simulink model "CC"  (R2015b)
settings: Solver=FixedStepDiscrete  StartTime=0.0  StopTime=inf  FixedStep=CCOk_stepSize  RelTol=1e-3
undefined symbols (not defined in the file or in its folder): CCOk_stepSize
settings Model: Creator=favv5g  LastModifiedBy=nctzv8
settings ConfigSet: Description=OpenECU configuration set for code generation under RTW-EC.
settings SolverCC: PositivePriorityOrder=on
settings DataIOCC: SaveFormat=Array  SignalLoggingSaveFormat=ModelDataLogs
settings OptimizationCC: DefaultParameterBehavior=Inlined  InlineInvariantSignals=on  ExpressionDepthLimit=2147483647  StateBitsets=on  DataBitsets=on  ZeroExternalMemoryAtStartup=off  ZeroInternalMemoryAtStartup=off  NoFixptDivByZeroProtection=on  EfficientFloat2IntCast=on  OptimizeModelRefInitCode=on  LifeSpan=1
settings DebuggingCC: SaveWithParameterizedLinksMsg=none  UnderspecifiedInitializationDetection=Classic  MergeDetectMultiDrivingBlocksExec=none  SignalResolutionControl=TryResolveAllWithWarning  MultiTaskDSMMsg=warning  MultiTaskCondExecSysMsg=none  SingleTaskRateTransMsg=error  CheckMatrixSingularityMsg=warning  VectorMatrixConversionMsg=warning  FcnCallInpInsideContextMsg=UseLocalSettings  SignalLabelMismatchMsg=warning  StateNameClashWarn=warning
settings HardwareCC: ProdBitPerPointer=32  ProdLargestAtomicInteger=Long  ProdLargestAtomicFloat=Double  ProdEndianess=BigEndian  ProdWordSize=32  ProdHWDeviceType=Freescale->32-bit PowerPC  TargetIntDivRoundTo=Zero  TargetEndianess=BigEndian  TargetHWDeviceType=Freescale->32-bit PowerPC  ProdEqTarget=off
settings RTWCC: SystemTargetFile=openecu_ert.tlc  MakeCommand=make_rtw optimized_floating_point=1  TemplateMakefile=openecu_ert_r2015b_64.tmf  Description=OpenECU Platform Target (ERT, optimised floating-point code)  RetainRTWFile=on  IncludeHyperlinkInReport=on
settings CodeAppCC: ForceParamTrailComments=on  IgnoreCustomStorageClasses=off  SimulinkDataObjDesc=on  CustomSymbolStrType=$N$R$M  InsertBlockDesc=on  InternalIdentifier=Classic
settings STFCustomTargetCC: TargetLibSuffix=.a  GenerateSampleERTMain=on  ConcurrentExecutionCompliant=off  IncludeMdlTerminateFcn=off  GeneratePreprocessorConditionals=Use local settings  CombineOutputUpdateFcns=on  IncludeFileDelimiter=UseQuote  ERTCustomFileBanners=on  SupportContinuousTime=off  MATLABClassNameForMDSCustomization=Simulink.SoftwareTarget.ERTCustomization  CPPClassGenCompliant=off  GRTInterface=off  SystemTargetFile=openecu_ert.tlc
settings ERTTargetCC: GenerateSampleERTMain=on  ParMdlRefBuildCompliant=off  CompOptLevelCompliant=off  ConcurrentExecutionCompliant=off  IncludeMdlTerminateFcn=off  ERTFirstTimeCompliant=off  IncludeFileDelimiter=UseQuote  SupportNonInlinedSFcns=on  ModelStepFunctionPrototypeControlCompliant=off  CPPClassGenCompliant=off  UseToolchainInfoCompliant=off  ExtModeMexFile=noextcomm  InlinedParameterPlacement=NonHierarchical  ERTSrcFileBannerTemplate=oe_code_c_template.cgt  ERTHdrFileBannerTemplate=oe_code_h_template.cgt  ERTDataSrcFileTemplate=oe_data_c_template.cgt  ERTDataHdrFileTemplate=oe_data_h_template.cgt  ERTCustomFileTemplate=example_file_process.tlc  GlobalDataDefinition=InSeparateSourceFile  GlobalDataReference=InSeparateHeaderFile  EnableUserReplacementTypes=on

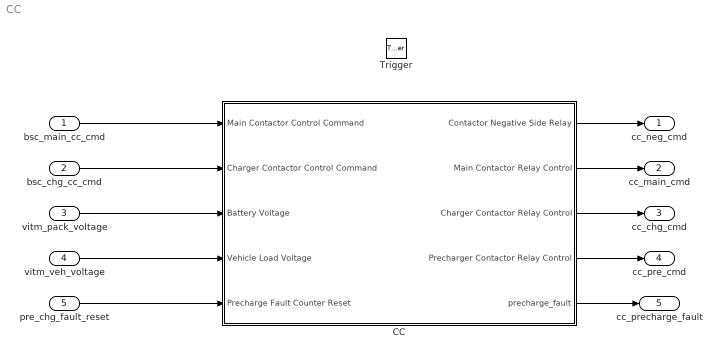
== system CC ==
  bsc_main_cc_cmd : Inport  OutDataTypeStr=boolean
  bsc_chg_cc_cmd : Inport  Port=2  OutDataTypeStr=boolean
  vitm_pack_voltage : Inport  Port=3
  vitm_veh_voltage : Inport  Port=4
  pre_chg_fault_reset : Inport  Port=5
  Trigger : TriggerPort  TriggerType=function-call  PortDimensions=1
  CC : Subsystem  TreatAsAtomicUnit=on
  cc_neg_cmd : Outport
  cc_main_cmd : Outport  Port=2
  cc_chg_cmd : Outport  Port=3
  cc_pre_cmd : Outport  Port=4
  cc_precharge_fault : Outport  Port=5
  wires:
  bsc_main_cc_cmd/1 -> CC/1(Main Contactor Control Command)
  bsc_chg_cc_cmd/1 -> CC/2(Charger Contactor Control Command)
  vitm_pack_voltage/1 -> CC/3(Battery Voltage)
  vitm_veh_voltage/1 -> CC/4(Vehicle Load Voltage)
  pre_chg_fault_reset/1 -> CC/5(Precharge Fault Counter Reset)
  CC/1("Contactor Negative Side Relay ") -> cc_neg_cmd/1
  CC/2("Main Contactor Relay Control ") -> cc_main_cmd/1
  CC/3(Charger Contactor Relay Control) -> cc_chg_cmd/1
  CC/4("Precharger Contactor Relay Control ") -> cc_pre_cmd/1
  CC/5(precharge_fault) -> cc_precharge_fault/1

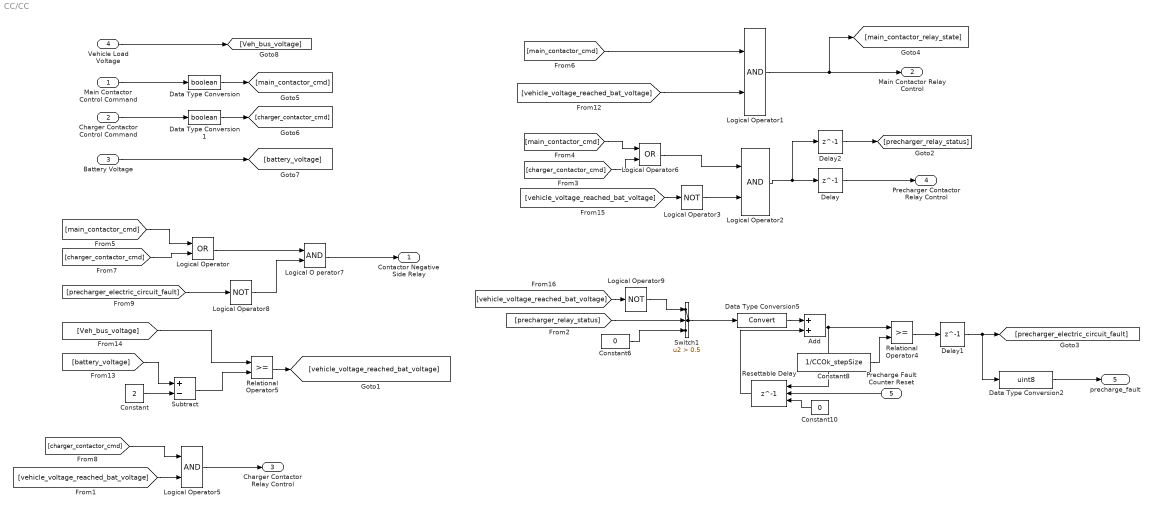
== system CC/CC ==
  Main Contactor Control Command : Inport  OutDataTypeStr=boolean
  Charger Contactor Control Command : Inport  Port=2  OutDataTypeStr=boolean
  Battery Voltage : Inport  Port=3
  Vehicle Load Voltage : Inport  Port=4
  Precharge Fault Counter Reset : Inport  Port=5
  Add : Sum  AccumDataTypeStr=uint16
  Constant : Constant  Value=2
  Constant10 : Constant  Value=0  OutDataTypeStr=Inherit: Inherit via back propagation
  Constant6 : Constant  Value=0
  Constant8 : Constant  Value=1/CCOk_stepSize  SampleTime=-1
  Data Type Conversion : DataTypeConversion  OutDataTypeStr=boolean
  Data Type Conversion1 : DataTypeConversion  OutDataTypeStr=boolean
  Data Type Conversion2 : DataTypeConversion  OutDataTypeStr=uint8
  Data Type Conversion5 : DataTypeConversion
  Delay : Delay  DelayLength=1
  Delay1 : Delay  DelayLength=1
  Delay2 : Delay  DelayLength=1
  Logical O perator7 : Logic  AllPortsSameDT=off  OutDataTypeStr=boolean
  Logical Operator : Logic  Operator=OR  AllPortsSameDT=off  OutDataTypeStr=boolean
  Logical Operator1 : Logic  AllPortsSameDT=off  OutDataTypeStr=boolean
  Logical Operator2 : Logic  AllPortsSameDT=off  OutDataTypeStr=boolean
  Logical Operator3 : Logic  Operator=NOT  AllPortsSameDT=off  OutDataTypeStr=boolean
  Logical Operator5 : Logic  AllPortsSameDT=off  OutDataTypeStr=boolean
  Logical Operator6 : Logic  Operator=OR  AllPortsSameDT=off  OutDataTypeStr=boolean
  Logical Operator8 : Logic  Operator=NOT  AllPortsSameDT=off  OutDataTypeStr=boolean
  Logical Operator9 : Logic  Operator=NOT  AllPortsSameDT=off  OutDataTypeStr=boolean
  Relational Operator4 : RelationalOperator  OutDataTypeStr=boolean
  Relational Operator5 : RelationalOperator  OutDataTypeStr=boolean
  Resettable Delay : Delay  DelayLength=1  InitialConditionSource=Input port  ExternalReset=Rising
      settings: InputPortMap=u0,r5,p4
  Subtract : Sum  Inputs=+-
  Switch1 : Switch  Criteria=u2 > Threshold  Threshold=0.5
  "Contactor Negative Side Relay " : Outport
  "Main Contactor Relay Control " : Outport  Port=2
  Charger Contactor Relay Control : Outport  Port=3
  "Precharger Contactor Relay Control " : Outport  Port=4
  precharge_fault : Outport  Port=5
  wires:
  Data Type Conversion1/1 -> [charger_contactor_cmd]
  Vehicle Load Voltage/1 -> [Veh_bus_voltage]
  [vehicle_voltage_reached_bat_voltage] -> Logical Operator9/1
  [battery_voltage] -> Subtract/1
  [vehicle_voltage_reached_bat_voltage] -> Logical Operator3/1
  Subtract/1 -> Relational Operator5/2
  Logical Operator9/1 -> Switch1/1
  Constant/1 -> Subtract/2
  Data Type Conversion2/1 -> precharge_fault/1
  Data Type Conversion/1 -> [main_contactor_cmd]
  [vehicle_voltage_reached_bat_voltage] -> Logical Operator1/2
  Precharge Fault Counter Reset/1 -> Resettable Delay/2
  Data Type Conversion5/1 -> Add/1
  Logical Operator5/1 -> Charger Contactor Relay Control/1
  [precharger_relay_status] -> Switch1/2
  Battery Voltage/1 -> [battery_voltage]
  Constant6/1 -> Switch1/3
  Add/1 -> Resettable Delay/1, Relational Operator4/1
  Switch1/1 -> Data Type Conversion5/1
  Relational Operator4/1 -> Delay1/1
  Constant10/1 -> Resettable Delay/3
  Constant8/1 -> Relational Operator4/2
  Delay1/1 -> Data Type Conversion2/1, [precharger_electric_circuit_fault]
  Resettable Delay/1 -> Add/2
  Logical O perator7/1 -> "Contactor Negative Side Relay "/1
  [main_contactor_cmd] -> Logical Operator/1
  [charger_contactor_cmd] -> Logical Operator/2
  Relational Operator5/1 -> [vehicle_voltage_reached_bat_voltage]
  [charger_contactor_cmd] -> Logical Operator5/1
  [main_contactor_cmd] -> Logical Operator1/1
  Logical Operator/1 -> Logical O perator7/1
  Logical Operator2/1 -> Delay/1, Delay2/1
  Logical Operator1/1 -> "Main Contactor Relay Control "/1, [main_contactor_relay_state]
  Charger Contactor Control Command/1 -> Data Type Conversion1/1
  [precharger_electric_circuit_fault] -> Logical Operator8/1
  Logical Operator8/1 -> Logical O perator7/2
  [Veh_bus_voltage] -> Relational Operator5/1
  Main Contactor Control Command/1 -> Data Type Conversion/1
  Logical Operator3/1 -> Logical Operator2/2
  [vehicle_voltage_reached_bat_voltage] -> Logical Operator5/2
  [main_contactor_cmd] -> Logical Operator6/1
  [charger_contactor_cmd] -> Logical Operator6/2
  Logical Operator6/1 -> Logical Operator2/1
  Delay/1 -> "Precharger Contactor Relay Control "/1
  Delay2/1 -> [precharger_relay_status]
